simulink model "Hilaire07"  (R2020b)
settings: Solver=ode3  StartTime=0.0  StopTime=t(end)  FixedStep=dt  RelTol=1e-3
values from neighbouring files (symbols this model uses):
  nInitial = initial_conditions(3)    [hilaire07martinez_simulink.m]    (also in jewett99_simulink.m)
  processLParams = [a0, p, beta, G, I0]    [hilaire07martinez_simulink.m]    (also in jewett99_simulink.m)
  processPParams = [mu, k, q, kc, tau]    [hilaire07martinez_simulink.m]    (also in jewett99_simulink.m)
  xInitial = [initial_conditions ... (first row only)    [gois09_simulink.m]    (also in hilaire07martinez_simulink.m = initial_conditions(1:2); jewett99_simulink.m = initial_conditions(1:2); ryzhii14_simulink.m; sinoatrial_simulink.m = initial_conditions)
undefined symbols (not defined in the file or in its folder): processNsParams
settings Model: Creator=chukw  LastModifiedBy=chukw

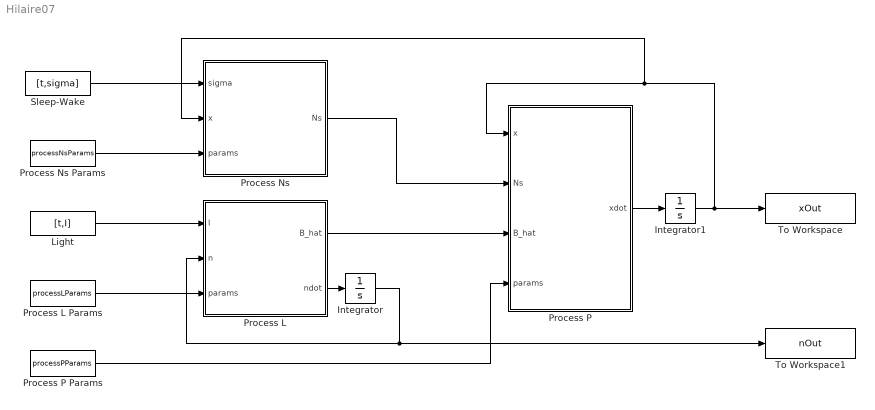
== system Hilaire07 ==
  Integrator : Integrator  InitialCondition=nInitial
  Integrator1 : Integrator  InitialCondition=xInitial
  Light : FromWorkspace  VariableName=[t,I]
  Process L : MATLAB Function  TreatAsAtomicUnit=on
  Process L Params : Constant  Value=processLParams
  Process Ns : MATLAB Function  TreatAsAtomicUnit=on
  Process Ns Params : Constant  Value=processNsParams
  Process P : MATLAB Function  TreatAsAtomicUnit=on
  Process P Params : Constant  Value=processPParams
  Sleep-Wake : FromWorkspace  VariableName=[t,sigma]
  To Workspace : ToWorkspace  VariableName=xOut  SampleTime=-1
  To Workspace1 : ToWorkspace  VariableName=nOut  SampleTime=-1
  wires:
  Integrator1/1 -> To Workspace/1, Process Ns/2(x), Process P/1(x)
  Process L/1(B_hat) -> Process P/3(B_hat)
  Process L Params/1 -> Process L/3(params)
  Process P Params/1 -> Process P/4(params)
  Integrator/1 -> Process L/2(n), To Workspace1/1
  Light/1 -> Process L/1(I)
  Process P/1(xdot) -> Integrator1/1
  Process L/2(ndot) -> Integrator/1
  Process Ns Params/1 -> Process Ns/3(params)
  Process Ns/1(Ns) -> Process P/2(Ns)
  Sleep-Wake/1 -> Process Ns/1(sigma)

== matlab function Hilaire07/Process P ==
  data: x input; Ns input; B_hat input; xdot output; params input
function xdot = processP(x,Ns,B_hat,params)

    mu = params(1);
    k = params(2);
    q = params(3);
    kc = params(4);
    tau = params(5);

    B = B_hat*(1-0.4*x(1))*(1-kc*x(2));

    xdot = zeros(2,1);
    xdot(1) = (pi/12)*(x(2) + mu*((x(1)/3)+(4*x(1)^3/3)-(256*x(1)^7/105)) + B + Ns);
    xdot(2) = (pi/12)*(q*x(2)*B - x(1)*( (24/0.99729/tau)^2 + k*B ));
end

== matlab function Hilaire07/Process L ==
  data: I input; B_hat output; n input; ndot output; params input
function [B_hat, ndot] = processL(I,n,params)

    a0 = params(1);
    p = params(2);
    Beta = params(3);
    G = params(4);
    I0 = params(5);
    
    alpha = (a0*(I/I0)^p) * (I/(I+100));
    ndot = 60*((alpha*(1-n)) - (Beta*n));
    B_hat = G*alpha*(1-n);
end

== matlab function Hilaire07/Process Ns ==
  data: sigma input; Ns output; x input; params input
function Ns  = processNs(sigma,x,params)
    rho = params(1);
    Ns_hat = rho*((1/3) - sigma);
    Ns = Ns_hat*(1 - tanh(10*x(1)));
end
